simulink model "multilevel_inverter"  (R2025b)
settings: Solver=FixedStepDiscrete  StartTime=0  StopTime=0.12  FixedStep=1e-6  RelTol=1e-3
libraries: spsIGBTDiodeLib x16, spsDCVoltageSourceLib x4, simulink x4, spsSeriesRLCBranchLib x2, spsVoltageMeasurementLib x2, spsCurrentMeasurementLib x1, sps_lib x1
settings Model: Creator=ASUS  LastModifiedBy=huy
settings DataIOCC: SaveFinalState=on  SaveOutput=off  SaveState=on  ReturnWorkspaceOutputs=off  LoggingToFile=on
settings RTWCC: GPUComputeCapability=3.5

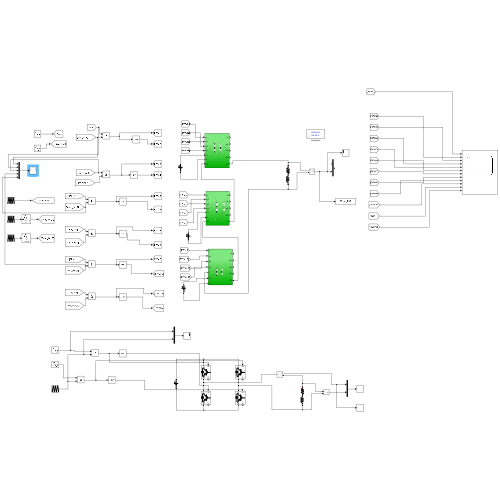
[thumbnail: Simulink's stored preview of the top-level diagram]
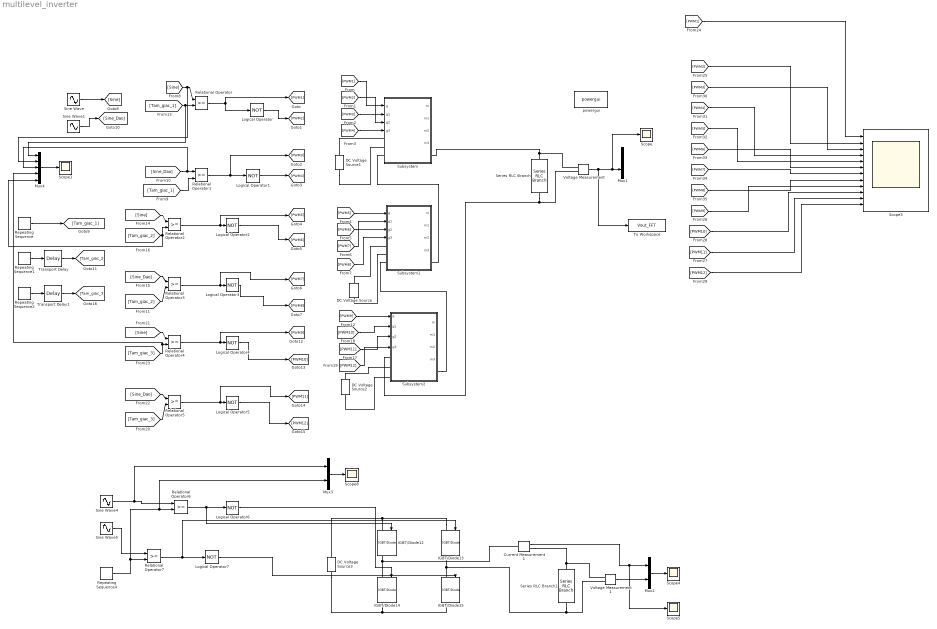
== system multilevel_inverter ==
  Current Measurement1 : spsCurrentMeasurementLib/Current Measurement  PhasorSimulation=off  OutputType=Complex  PSBequivalent=0
  DC Voltage Source : spsDCVoltageSourceLib/DC Voltage Source  Amplitude=12  Measurements=None
  DC Voltage Source1 : spsDCVoltageSourceLib/DC Voltage Source  Amplitude=12  Measurements=None
  DC Voltage Source2 : spsDCVoltageSourceLib/DC Voltage Source  Amplitude=12  Measurements=None
  DC Voltage Source3 : spsDCVoltageSourceLib/DC Voltage Source  Amplitude=100  Measurements=None
  IGBT/Diode{12..15} (4 alike) : spsIGBTDiodeLib/IGBT//Diode  Ron=1e-3  Rs=1e5  Cs=inf  Measurements=on
  Logical Operator{,1..7} (8 alike) : Logic  Operator=NOT  AllPortsSameDT=off  OutDataTypeStr=boolean
  Mux1 : Mux  Inputs=2
  Mux2 : Mux  Inputs=2
  Mux3 : Mux  Inputs=2
  Mux4 : Mux  Inputs=5
  Relational Operator{,1..7} (8 alike) : RelationalOperator  OutDataTypeStr=boolean  RndMeth=Simplest  InputSameDT=off
  Repeating Sequence : simulink/Sources/Repeating Sequence  rep_seq_t=[0 0.5 1]/25595  rep_seq_y=[-1 1 -1]
  Repeating Sequence1 : simulink/Sources/Repeating Sequence  rep_seq_t=[0 0.5 1]/25595  rep_seq_y=[-1 1 -1]
  Repeating Sequence2 : simulink/Sources/Repeating Sequence  rep_seq_t=[0 0.5 1]/25595  rep_seq_y=[-1 1 -1]
  Repeating Sequence4 : simulink/Sources/Repeating Sequence  rep_seq_t=[0 0.5 1]/25056  rep_seq_y=[-1 1 -1]
  Scope{,1,4..5,8} (5 alike) : Scope
      Scope settings: Title=DẠNG SÓNG ĐIỆN ÁP AC 7 BẬC  ActiveDisplayYMinimum=-45.595846303696163  ActiveDisplayYMaximum=44.362191426003307  YLabel=Volts  DataLoggingVariableName=Data_output
      Scope1 settings: Title=SÓNG TAM GIÁC DỊCH PHA VÀ SÓNG SINE  ActiveDisplayYMinimum=-1.328107126323504  ActiveDisplayYMaximum=1.2708580809087289  YLabel=BIÊN ĐỘ  DataLoggingVariableName=Data_output1
      Scope4 settings: ActiveDisplayYMinimum=-95.3901241808319  ActiveDisplayYMaximum=126.36935234163921  DataLoggingVariableName=Data_Output1
      Scope5 settings: ActiveDisplayYMinimum=-72.4010073201923  ActiveDisplayYMaximum=72.404345691734761
      Scope8 settings: ActiveDisplayYMinimum=-1.2842668623835931  ActiveDisplayYMaximum=1.2150931376152658  DataLoggingVariableName=Data_Output3
  Scope3 : Scope  NumInputPorts=12
      settings: ActiveDisplayYMinimum=-0.01914531422513277  ActiveDisplayYMaximum=1.0428513200142151  DataLoggingVariableName=ScopeData3
  Series RLC Branch : spsSeriesRLCBranchLib/Series RLC Branch  LConnTagsString=__new0  RConnTagsString=__new0  BranchType=RL  Resistance=5  Inductance=5e-3  SetiL0=off  InitialCurrent=0  Capacitance=1e-6  Setx0=off  InitialVoltage=0  Measurements=None
  Series RLC Branch1 : spsSeriesRLCBranchLib/Series RLC Branch  LConnTagsString=__new0  RConnTagsString=__new0  BranchType=RL  Resistance=5  Inductance=5e-3  SetiL0=off  InitialCurrent=0  Capacitance=1e-6  Setx0=off  InitialVoltage=0  Measurements=None
  Sine Wave : Sin  Amplitude=0.96  Frequency=2*pi*50  SampleTime=0
  Sine Wave1 : Sin  Amplitude=-0.96  Frequency=2*pi*50  SampleTime=0
  Sine Wave4 : Sin  Amplitude=0.9  Frequency=2*pi*50  SampleTime=0
  Sine Wave5 : Sin  Amplitude=-0.9  Frequency=2*pi*50  SampleTime=0
  Subsystem : Subsystem
  Subsystem1 : Subsystem
  Subsystem2 : Subsystem
  To Workspace : ToWorkspace  VariableName=Vout_FFT  SaveFormat=Structure  SampleTime=-1
  Transport Delay : TransportDelay  DelayTime=(1/25595)*(60/360)
  Transport Delay1 : TransportDelay  DelayTime=(1/25595)*(60/360)*2
  Voltage Measurement : spsVoltageMeasurementLib/Voltage Measurement  PhasorSimulation=off  OutputType=Complex  PSBequivalent=0
  Voltage Measurement1 : spsVoltageMeasurementLib/Voltage Measurement  PhasorSimulation=off  OutputType=Complex  PSBequivalent=0
  powergui : sps_lib/powergui  Priority=1  SimulationMode=Discrete  SampleTime=50e-6  frequency=60  Iterations=50  frequencyindice=0  Pbase=100e6  ErrMax=1e-4  UnitsV=kV  UnitsW=MW  buscounter=0  FunctionMessages=off  echomessages=off  EnableUseOfTLC=off  CurrentSourceSwitches=off  DisableSnubberDevices=off  DisableRonSwitches=off  DisableVfSwitches=off  DisplayEquations=off  AutomaticDiscreteSolvers=off  SolverType=Tustin/Backward Euler (TBE)  Interpol=off  ExternalGateDelay=off  methode=off  Ts=100  x0status=blocks  SPID=on  SwTol=0  HookPort=off  NonlinearTolerance=1e-4  nMaxIteration=100  ContinueOnMaxIteration=off  RestoreLinks=warning  ResistiveCurrentMeasurement=off  Frange=[0:2:500]  Ylog=off  Xlog=on  ShowGrid=off  save=off  variable=ZData  structure=0  ZoomFFT=off  StartTime=0.0  cycles=1  DisplayStyle=1  fundamental=60  FreqAxis=off  MaxFrequency=1000  frequencyindicesteady=1  RmsSteady=1  display=off
  wires:
  Sine Wave/1 -> [Sine]
  Relational Operator/1 -> [PWM1], Logical Operator/1
  Relational Operator1/1 -> [PWM3], Logical Operator1/1
  Repeating Sequence/1 -> [Tam_giac_1]
  Sine Wave1/1 -> [Sine_Dao]
  Logical Operator/1 -> [PWM2]
  Logical Operator1/1 -> [PWM4]
  Repeating Sequence1/1 -> Transport Delay/1
  Transport Delay/1 -> [Tam_giac_2]
  Relational Operator2/1 -> [PWM5], Logical Operator2/1
  Relational Operator3/1 -> [PWM7], Logical Operator3/1
  Logical Operator2/1 -> [PWM6]
  Logical Operator3/1 -> [PWM8]
  [Sine] -> Mux4/2, Relational Operator/1
  [Tam_giac_1] -> Mux4/1, Relational Operator/2
  [Tam_giac_1] -> Relational Operator1/2
  [Sine] -> Relational Operator2/1
  [Sine_Dao] -> Mux4/3, Relational Operator1/1
  [Sine_Dao] -> Relational Operator3/1
  [Tam_giac_2] -> Relational Operator3/2
  [Tam_giac_2] -> Relational Operator2/2, Mux4/5
  [Sine] -> Relational Operator4/1
  [Sine_Dao] -> Relational Operator5/1
  Logical Operator4/1 -> [PWM10]
  [Tam_giac_3] -> Mux4/4, Relational Operator4/2
  [Tam_giac_3] -> Relational Operator5/2
  Logical Operator5/1 -> [PWM12]
  Relational Operator5/1 -> [PWM11], Logical Operator5/1
  Relational Operator4/1 -> [PWM9], Logical Operator4/1
  Transport Delay1/1 -> [Tam_giac_3]
  Repeating Sequence2/1 -> Transport Delay1/1
  [PWM1] -> Scope3/1
  [PWM2] -> Scope3/2
  [PWM3] -> Scope3/3
  [PWM4] -> Scope3/4
  [PWM5] -> Scope3/5
  [PWM6] -> Scope3/6
  [PWM7] -> Scope3/7
  [PWM8] -> Scope3/8
  [PWM9] -> Scope3/9
  [PWM10] -> Scope3/10
  [PWM11] -> Scope3/11
  [PWM12] -> Scope3/12
  Relational Operator7/1 -> IGBT/Diode13/1, Logical Operator7/1
  Logical Operator7/1 -> IGBT/Diode15/1
  Relational Operator6/1 -> IGBT/Diode12/1, Logical Operator6/1
  Logical Operator6/1 -> IGBT/Diode14/1
  Mux2/1 -> Scope4/1
  Current Measurement1/1 -> Mux2/1, Scope5/1
  Voltage Measurement1/1 -> Mux2/2
  Sine Wave5/1 -> Relational Operator7/1
  Repeating Sequence4/1 -> Relational Operator7/2, Mux3/2, Relational Operator6/2
  Sine Wave4/1 -> Mux3/1, Relational Operator6/1
  Mux3/1 -> Scope8/1
  Voltage Measurement/1 -> To Workspace/1, Scope/1, Mux1/2
  [PWM1] -> Subsystem/1(g)
  [PWM3] -> Subsystem/2(g1)
  [PWM2] -> Subsystem/3(g2)
  [PWM4] -> Subsystem/4(g3)
  [PWM5] -> Subsystem1/1(g)
  [PWM7] -> Subsystem1/2(g1)
  [PWM6] -> Subsystem1/3(g2)
  [PWM8] -> Subsystem1/4(g3)
  [PWM9] -> Subsystem2/1(g)
  [PWM10] -> Subsystem2/2(g1)
  [PWM11] -> Subsystem2/3(g2)
  [PWM12] -> Subsystem2/4(g3)
  Mux4/1 -> Scope1/1
  connections:
  Series RLC Branch/RConn1 -- Subsystem2/LConn1 -- Voltage Measurement/LConn2
  Voltage Measurement/LConn1 -- Subsystem/RConn1 -- Series RLC Branch/LConn1
  IGBT/Diode12/RConn1 -- IGBT/Diode14/LConn1 -- Current Measurement1/LConn1
  Series RLC Branch1/RConn1 -- IGBT/Diode15/LConn1 -- IGBT/Diode13/RConn1 -- Voltage Measurement1/LConn2
  IGBT/Diode15/RConn1 -- DC Voltage Source3/LConn1 -- IGBT/Diode14/RConn1
  IGBT/Diode13/LConn1 -- DC Voltage Source3/RConn1 -- IGBT/Diode12/LConn1
  Series RLC Branch1/LConn1 -- Current Measurement1/RConn1 -- Voltage Measurement1/LConn1
  DC Voltage Source1/RConn1 -- Subsystem/LConn1
  DC Voltage Source1/LConn1 -- Subsystem/LConn2
  Subsystem/LConn3 -- Subsystem1/RConn1
  DC Voltage Source/RConn1 -- Subsystem1/LConn1
  Subsystem1/LConn2 -- DC Voltage Source/LConn1
  Subsystem2/RConn1 -- Subsystem1/LConn3
  DC Voltage Source2/RConn1 -- Subsystem2/LConn2
  Subsystem2/LConn3 -- DC Voltage Source2/LConn1

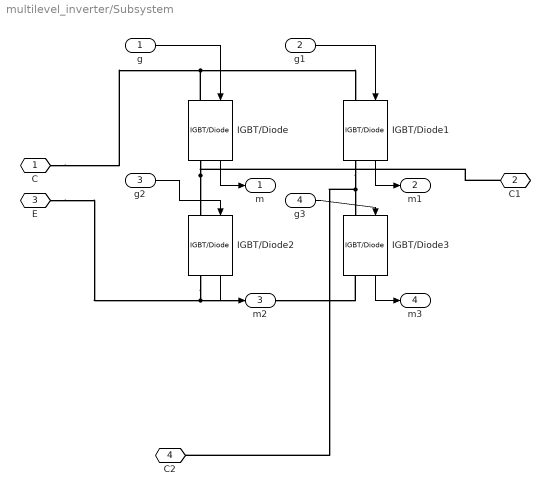
== system multilevel_inverter/Subsystem ==
  g : Inport
  g1 : Inport  Port=2
  g2 : Inport  Port=3
  g3 : Inport  Port=4
  IGBT/Diode{,1..3} (4 alike) : spsIGBTDiodeLib/IGBT//Diode  Ron=1e-3  Rs=1e5  Cs=inf  Measurements=on
  C : PMIOPort  Side=Left
  C1 : PMIOPort  Port=2  Side=Right
  E : PMIOPort  Port=3  Side=Left
  C2 : PMIOPort  Port=4  Side=Left
  m : Outport
  m1 : Outport  Port=2
  m2 : Outport  Port=3
  m3 : Outport  Port=4
  wires:
  IGBT/Diode2/1 -> m2/1
  IGBT/Diode3/1 -> m3/1
  g1/1 -> IGBT/Diode1/1
  g3/1 -> IGBT/Diode3/1
  g/1 -> IGBT/Diode/1
  IGBT/Diode/1 -> m/1
  IGBT/Diode1/1 -> m1/1
  g2/1 -> IGBT/Diode2/1
  connections:
  IGBT/Diode1/RConn1 -- C2/RConn1 -- IGBT/Diode3/LConn1
  IGBT/Diode/RConn1 -- IGBT/Diode2/LConn1 -- C1/RConn1
  IGBT/Diode/LConn1 -- C/RConn1 -- IGBT/Diode1/LConn1
  IGBT/Diode2/RConn1 -- E/RConn1 -- IGBT/Diode3/RConn1

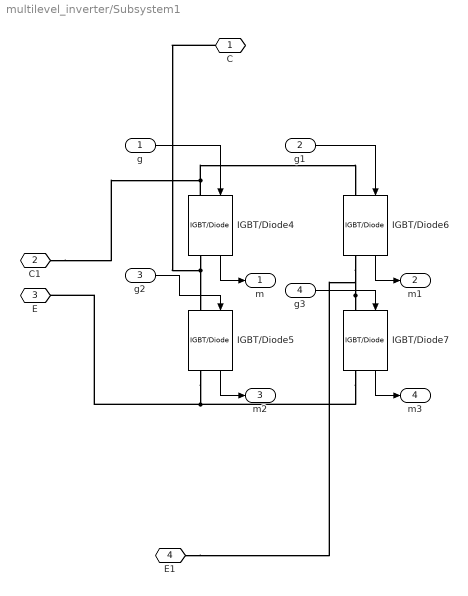
== system multilevel_inverter/Subsystem1 ==
  g : Inport
  g1 : Inport  Port=2
  g2 : Inport  Port=3
  g3 : Inport  Port=4
  IGBT/Diode{4..7} (4 alike) : spsIGBTDiodeLib/IGBT//Diode  Ron=1e-3  Rs=1e5  Cs=inf  Measurements=on
  C : PMIOPort  Side=Right
  C1 : PMIOPort  Port=2  Side=Left
  E : PMIOPort  Port=3  Side=Left
  E1 : PMIOPort  Port=4  Side=Left
  m : Outport
  m1 : Outport  Port=2
  m2 : Outport  Port=3
  m3 : Outport  Port=4
  wires:
  IGBT/Diode6/1 -> m1/1
  IGBT/Diode4/1 -> m/1
  IGBT/Diode7/1 -> m3/1
  g2/1 -> IGBT/Diode5/1
  g1/1 -> IGBT/Diode6/1
  IGBT/Diode5/1 -> m2/1
  g3/1 -> IGBT/Diode7/1
  g/1 -> IGBT/Diode4/1
  connections:
  IGBT/Diode4/RConn1 -- C/RConn1 -- IGBT/Diode5/LConn1
  IGBT/Diode7/LConn1 -- E1/RConn1 -- IGBT/Diode6/RConn1
  IGBT/Diode4/LConn1 -- IGBT/Diode6/LConn1 -- C1/RConn1
  IGBT/Diode7/RConn1 -- E/RConn1 -- IGBT/Diode5/RConn1

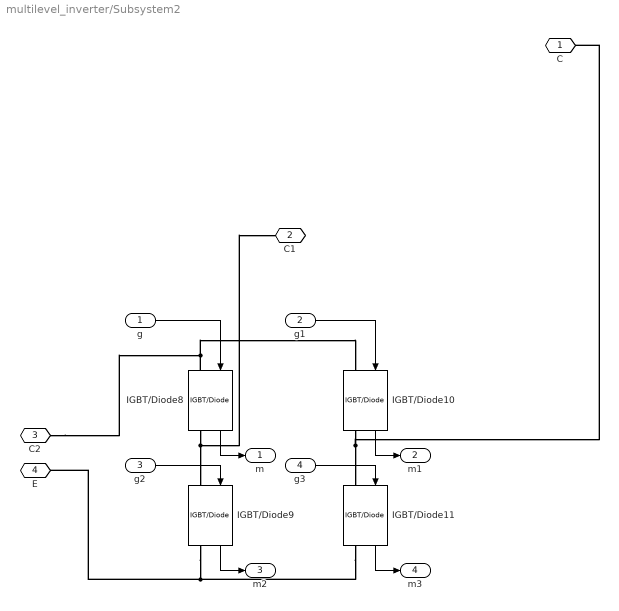
== system multilevel_inverter/Subsystem2 ==
  g : Inport
  g1 : Inport  Port=2
  g2 : Inport  Port=3
  g3 : Inport  Port=4
  IGBT/Diode{8..11} (4 alike) : spsIGBTDiodeLib/IGBT//Diode  Ron=1e-3  Rs=1e5  Cs=inf  Measurements=on
  C : PMIOPort  Side=Left
  C1 : PMIOPort  Port=2  Side=Right
  C2 : PMIOPort  Port=3  Side=Left
  E : PMIOPort  Port=4  Side=Left
  m : Outport
  m1 : Outport  Port=2
  m2 : Outport  Port=3
  m3 : Outport  Port=4
  wires:
  IGBT/Diode11/1 -> m3/1
  IGBT/Diode9/1 -> m2/1
  IGBT/Diode10/1 -> m1/1
  g/1 -> IGBT/Diode8/1
  g1/1 -> IGBT/Diode10/1
  IGBT/Diode8/1 -> m/1
  g2/1 -> IGBT/Diode9/1
  g3/1 -> IGBT/Diode11/1
  connections:
  IGBT/Diode8/RConn1 -- C1/RConn1 -- IGBT/Diode9/LConn1
  IGBT/Diode11/RConn1 -- E/RConn1 -- IGBT/Diode9/RConn1
  IGBT/Diode8/LConn1 -- IGBT/Diode10/LConn1 -- C2/RConn1
  IGBT/Diode10/RConn1 -- IGBT/Diode11/LConn1 -- C/RConn1
